simulink model "question3"  (R2023b)
settings: Solver=VariableStepAuto  StartTime=0.0  StopTime=10.0  RelTol=1e-3
values from neighbouring files (symbols this model uses):
  A = [-8.8487+(a-b)/5,-0.0399,-5.55+(c+d)/10,3.5846 ... (first row only)    [main_func.m]    (also in question3.m = [-8.8487+(a-b)/5, -0.0399, -5.55+(c+d)/10, 3.5846)
  B = [0.0564+b/(10+c),0.0319 ... (first row only)    [main_func.m]    (also in question3.m = [0.0564+b/(10+c), 0.0319)
  C = [-3.2988,-2.1932+(10*c+d)/(100+5*a),0.037,-0.0109 ... (first row only)    [main_func.m]    (also in question3.m = [-3.2988, -2.1932+(10*c+d)/(100+5*a), 0.037, -0.0109)
  K2 = lqr(A,B,Q,R)    [main_func.m]    (also in servo_control.m = K(:,5:6); servo_control_state.m = K(:,5:6))
  L = L'    [main_func.m]    (also in question3.m = place(A', C', observer_poles)'; servo_control.m)
  x0 = [0.5;-0.1;0.3;-0.8]    [main_func.m]    (also in question3.m = [0.5; -0.1; 0.3; -0.8])
settings Model: Creator=Fan Xiuqi  LastModifiedBy=Fan Xiuqi

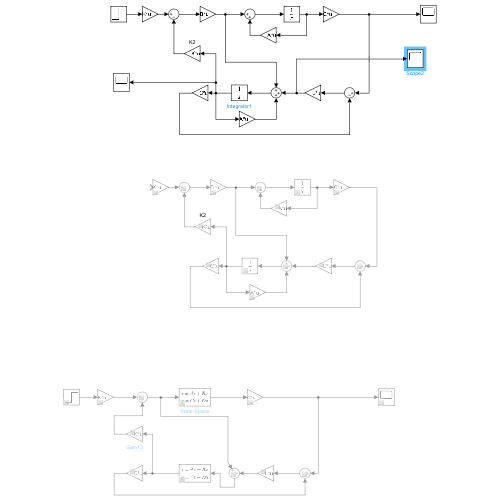
[thumbnail: Simulink's stored preview of the top-level diagram]
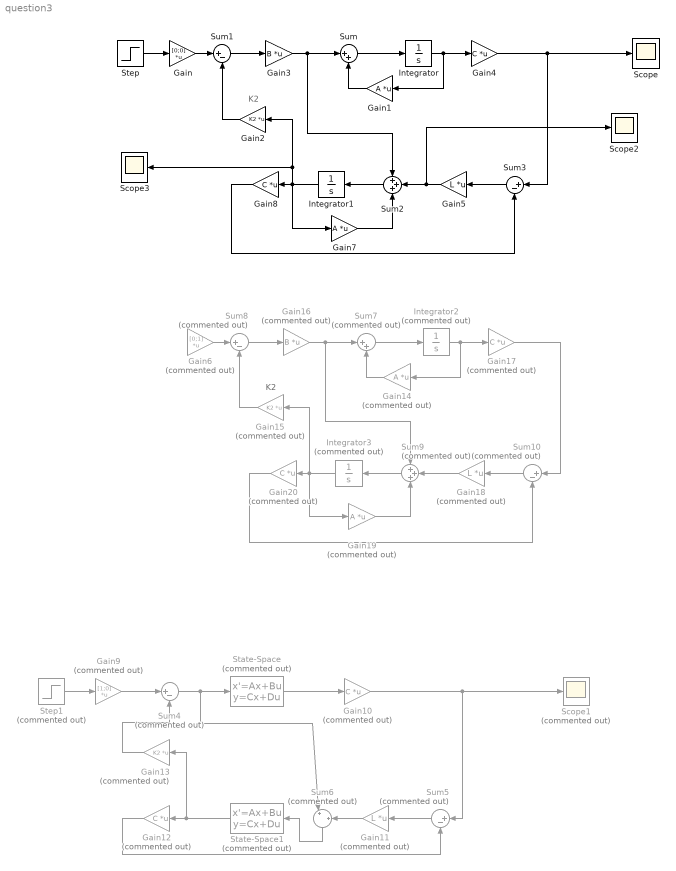
== system question3 ==
  note: K2
  note: K2
  Gain : Gain  Gain=[0;0]  Multiplication=Matrix(K*u)
  Gain1 : Gain  Gain=A  Multiplication=Matrix(K*u)
  Gain{10,12,17,20} (4 alike) : Gain  Commented=on  Gain=C  Multiplication=Matrix(K*u)
  Gain11 : Gain  Commented=on  Gain=L  Multiplication=Matrix(K*u)
  Gain13 : Gain  Commented=on  Gain=K2  Multiplication=Matrix(K*u)
  Gain14 : Gain  Commented=on  Gain=A  Multiplication=Matrix(K*u)
  Gain15 : Gain  Commented=on  Gain=K2  Multiplication=Matrix(K*u)
  Gain16 : Gain  Commented=on  Gain=B  Multiplication=Matrix(K*u)
  Gain18 : Gain  Commented=on  Gain=L  Multiplication=Matrix(K*u)
  Gain19 : Gain  Commented=on  Gain=A  Multiplication=Matrix(K*u)
  Gain2 : Gain  Gain=K2  Multiplication=Matrix(K*u)
  Gain3 : Gain  Gain=B  Multiplication=Matrix(K*u)
  Gain4 : Gain  Gain=C  Multiplication=Matrix(K*u)
  Gain5 : Gain  Gain=L  Multiplication=Matrix(K*u)
  Gain6 : Gain  Commented=on  Gain=[0;1]  Multiplication=Matrix(K*u)
  Gain7 : Gain  Gain=A  Multiplication=Matrix(K*u)
  Gain8 : Gain  Gain=C  Multiplication=Matrix(K*u)
  Gain9 : Gain  Commented=on  Gain=[1;0]  Multiplication=Matrix(K*u)
  Integrator : Integrator  InitialCondition=x0
  Integrator1 : Integrator  InitialCondition=x0
  Integrator2 : Integrator  Commented=on
  Integrator3 : Integrator  Commented=on
  Scope : Scope
  Scope1 : Scope  Commented=on
  Scope2 : Scope
  Scope3 : Scope
  State-Space : StateSpace  Commented=on  A=A  B=B  C=eye(4)  D=zeros(4,2)  InitialCondition=0
  State-Space1 : StateSpace  Commented=on  A=A  B=B  C=eye(4)  D=zeros(4,2)  InitialCondition=0
  Step : Step  SampleTime=0
  Step1 : Step  Commented=on  SampleTime=0
  Sum : Sum  Inputs=|++
  Sum1 : Sum  Inputs=|+-
  Sum{4..5,8,10} (4 alike) : Sum  Commented=on  Inputs=|+-
  Sum2 : Sum  Inputs=+++
  Sum3 : Sum  Inputs=|+-
  Sum6 : Sum  Commented=on  Inputs=|+|+
  Sum7 : Sum  Commented=on  Inputs=|++
  Sum9 : Sum  Commented=on  Inputs=+++
  wires:
  Step/1 -> Gain/1
  Gain1/1 -> Sum/2
  Integrator/1 -> Gain1/1, Gain4/1
  Gain3/1 -> Sum/1, Sum2/1
  Sum/1 -> Integrator/1
  Sum1/1 -> Gain3/1
  Gain/1 -> Sum1/1
  Sum2/1 -> Integrator1/1
  Gain5/1 -> Scope2/1, Sum2/2
  Integrator1/1 -> Gain7/1, Scope3/1, Gain2/1, Gain8/1
  Gain7/1 -> Sum2/3
  Sum3/1 -> Gain5/1
  Gain4/1 -> Sum3/1, Scope/1
  Gain8/1 -> Sum3/2
  Gain2/1 -> Sum1/2
  Step1/1 -> Gain9/1
  Gain9/1 -> Sum4/1
  Sum4/1 -> Sum6/1, State-Space/1
  State-Space/1 -> Gain10/1
  Gain10/1 -> Scope1/1, Sum5/1
  Sum5/1 -> Gain11/1
  State-Space1/1 -> Gain13/1, Gain12/1
  Gain12/1 -> Sum5/2
  Gain13/1 -> Sum4/2
  Gain11/1 -> Sum6/2
  Sum6/1 -> State-Space1/1
  Sum8/1 -> Gain16/1
  Gain16/1 -> Sum7/1, Sum9/1
  Gain6/1 -> Sum8/1
  Gain15/1 -> Sum8/2
  Gain17/1 -> Sum10/1
  Integrator3/1 -> Gain19/1, Gain15/1, Gain20/1
  Sum10/1 -> Gain18/1
  Gain14/1 -> Sum7/2
  Gain18/1 -> Sum9/2
  Gain20/1 -> Sum10/2
  Gain19/1 -> Sum9/3
  Sum7/1 -> Integrator2/1
  Sum9/1 -> Integrator3/1
  Integrator2/1 -> Gain14/1, Gain17/1
